simulink model "ATTITUDE_DETERMINATION"  (R2024b)
settings: Solver=VariableStepAuto  StartTime=0.0  StopTime=10.0  RelTol=1e-3
libraries: matrix_library x7
settings Model: Creator=esteb  LastModifiedBy=esteb

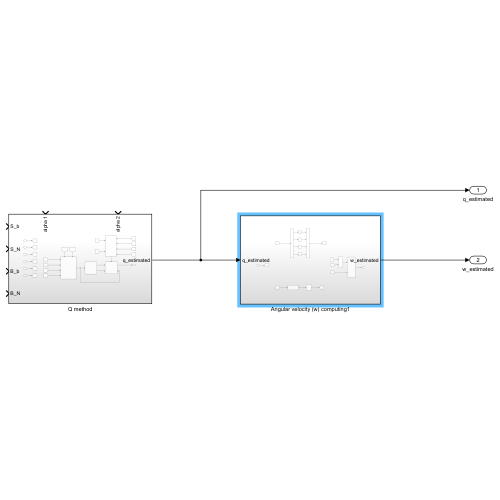
[thumbnail: Simulink's stored preview of the top-level diagram]
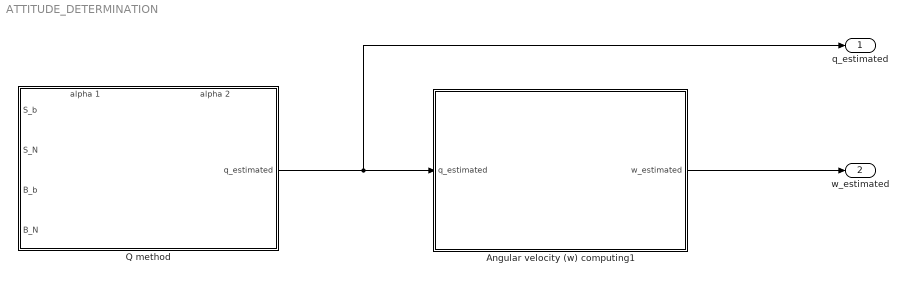
== system ATTITUDE_DETERMINATION ==
  Angular velocity (w) computing1 : Subsystem
  Q method : Subsystem
      settings: PortSchema="{\"entries\":[{\"content\":{\"sides\":[{\"content\":{\"connectorIds\":[\"In1\",\"In2\",\"In3\",\"In4\"]},\"type\":\"ConnectorPlacement.EquallySpacedRectSide\",\"uuid\":\"15956c10-3c30-4cb4-a63c-f434daa5cd48\"},{\"content\":{\"connectorIds\":[\"Out1\"],\"side\":\"RIGHT\"},\"type\":\"ConnectorPlacement.EquallySpacedRectSide\",\"uuid\":\"3f26d307-35c8-43a0-9998-86e1286678fb\"},{\"content\":{\"connectorIds\":[\"In5\",\"In6\"],\"side\":\"TOP\"},\"type\":\"ConnectorPlacement.EquallySpacedRectSide\",\"uuid\":\"55f51305-766e-4e3f-8617-95c7676083b2\"}]},\"type\":\"ConnectorPlacement.EquallySpacedConnector\",\"uuid\":\"09b6cbb7-0430-4316-92af-7ec4423129aa\"}],\"packageUris\":[\"http://schema.mathworks.com/mf0/Connector/R2020b\"],\"version\":\"1.0\"}"
  q_estimated : Outport
  w_estimated : Outport  Port=2
  wires:
  Q method/1(q_estimated) -> Angular velocity (w) computing1/1(q_estimated), q_estimated/1
  Angular velocity (w) computing1/1(w_estimated) -> w_estimated/1

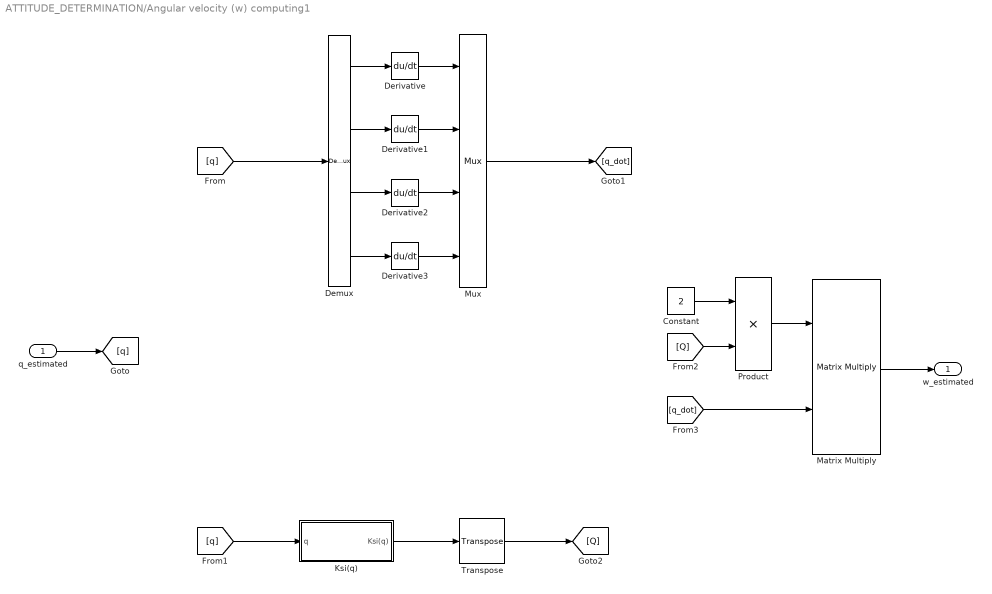
== system ATTITUDE_DETERMINATION/Angular velocity (w) computing1 ==
  q_estimated : Inport
  Constant : Constant  Value=2
  Demux : Demux
  Derivative{,1..3} (4 alike) : Derivative
  Ksi(q) : Subsystem
  Matrix Multiply : Product  Multiplication=Matrix(*)
  Mux : Mux
  Product : Product
  Transpose : matrix_library/Transpose
  w_estimated : Outport
  wires:
  q_estimated/1 -> [q]
  [q] -> Demux/1
  Demux/1 -> Derivative/1
  Demux/2 -> Derivative1/1
  Demux/3 -> Derivative2/1
  Demux/4 -> Derivative3/1
  [q] -> Ksi(q)/1(q)
  Mux/1 -> [q_dot]
  [Q] -> Product/2
  Constant/1 -> Product/1
  [q_dot] -> Matrix Multiply/2
  Matrix Multiply/1 -> w_estimated/1
  Derivative/1 -> Mux/1
  Derivative1/1 -> Mux/2
  Derivative2/1 -> Mux/3
  Derivative3/1 -> Mux/4
  Product/1 -> Matrix Multiply/1
  Ksi(q)/1(Ksi(q)) -> Transpose/1
  Transpose/1 -> [Q]

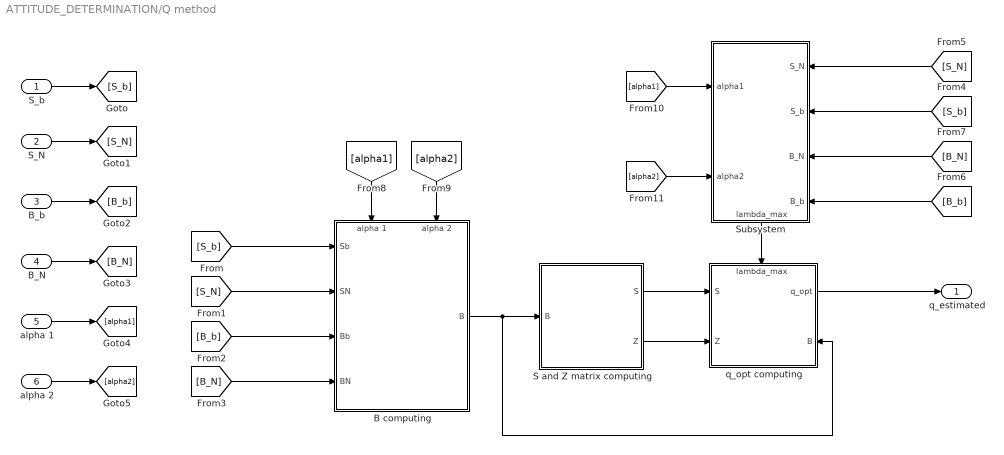
== system ATTITUDE_DETERMINATION/Q method ==
  S_b : Inport
  S_N : Inport  Port=2
  B_b : Inport  Port=3
  B_N : Inport  Port=4
  alpha 1 : Inport  Port=5
  alpha 2 : Inport  Port=6
  B computing : Subsystem
      settings: PortSchema="{\"entries\":[{\"content\":{\"sides\":[{\"content\":{\"connectorIds\":[\"In1\",\"In2\",\"In3\",\"In4\"]},\"type\":\"ConnectorPlacement.EquallySpacedRectSide\",\"uuid\":\"50fc9399-82b5-4b10-921b-f93011029ce3\"},{\"content\":{\"connectorIds\":[\"Out1\"],\"side\":\"RIGHT\"},\"type\":\"ConnectorPlacement.EquallySpacedRectSide\",\"uuid\":\"3981c554-ab38-4f62-9b84-94877d1cd2ff\"},{\"content\":{\"connectorIds\":[\"In5\",\"In6\"],\"side\":\"TOP\"},\"type\":\"ConnectorPlacement.EquallySpacedRectSide\",\"uuid\":\"ba062d99-6f44-4068-8114-c0cfa81f1ff2\"},{\"content\":{\"side\":\"BOTTOM\"},\"type\":\"ConnectorPlacement.EquallySpacedRectSide\",\"uuid\":\"0ce0d8e8-da8b-4b2d-90df-7b0bc851bc5b\"}]},\"type\":\"ConnectorPlacement.EquallySpacedConnector\",\"uuid\":\"bcda7430-c6c8-4f59-a99a-b367d20ffcb5\"}],\"packageUris\":[\"http://schema.mathworks.com/mf0/Connector/R2020b\"],\"version\":\"1.0\"}"
  S and Z matrix computing : Subsystem
  Subsystem : Subsystem
      settings: PortSchema="{\"entries\":[{\"content\":{\"sides\":[{\"content\":{\"connectorIds\":[\"Out1\"]},\"type\":\"ConnectorPlacement.EquallySpacedRectSide\",\"uuid\":\"5768cb62-7f28-4cce-8da1-dcdd14add895\"},{\"content\":{\"side\":\"RIGHT\"},\"type\":\"ConnectorPlacement.EquallySpacedRectSide\",\"uuid\":\"8778aa17-5802-4f6c-9df9-b85455c7c074\"},{\"content\":{\"connectorIds\":[\"In1\",\"In2\"],\"side\":\"TOP\"},\"type\":\"ConnectorPlacement.EquallySpacedRectSide\",\"uuid\":\"8a3cb844-269f-4d3f-b8ee-2af4584390c1\"},{\"content\":{\"connectorIds\":[\"In3\",\"In4\",\"In5\",\"In6\"],\"side\":\"BOTTOM\"},\"type\":\"ConnectorPlacement.EquallySpacedRectSide\",\"uuid\":\"ccc3bad4-265e-44f4-a8b0-aae769a28e60\"}]},\"type\":\"ConnectorPlacement.EquallySpacedConnector\",\"uuid\":\"9389ccda-4d08-49a8-9951-bd9019203c57\"}],\"packageUris\":[\"http://schema.mathworks.com/mf0/Connector/R2020b\"],\"version\":\"1.0\"}"
  q_opt computing : Subsystem
      settings: PortSchema="{\"entries\":[{\"content\":{\"sides\":[{\"content\":{\"connectorIds\":[\"In1\",\"In2\"]},\"type\":\"ConnectorPlacement.EquallySpacedRectSide\",\"uuid\":\"077e0174-8a2c-4f76-bac9-e91df836f5e1\"},{\"content\":{\"connectorIds\":[\"Out1\",\"In4\"],\"side\":\"RIGHT\"},\"type\":\"ConnectorPlacement.EquallySpacedRectSide\",\"uuid\":\"0e923535-8f32-4607-bd4a-42896d211835\"},{\"content\":{\"connectorIds\":[\"In3\"],\"side\":\"TOP\"},\"type\":\"ConnectorPlacement.EquallySpacedRectSide\",\"uuid\":\"91682e2a-1ae8-44b6-9458-d5d75f2c9b10\"},{\"content\":{\"side\":\"BOTTOM\"},\"type\":\"ConnectorPlacement.EquallySpacedRectSide\",\"uuid\":\"ebee2d10-c6a3-420b-a3da-5d4d259a0e4d\"}]},\"type\":\"ConnectorPlacement.EquallySpacedConnector\",\"uuid\":\"6651e596-192f-4f32-9855-13a8c081df01\"}],\"packageUris\":[\"http://schema.mathworks.com/mf0/Connector/R2020b\"],\"version\":\"1.0\"}"
  q_estimated : Outport
  wires:
  [alpha2] -> Subsystem/1(alpha2)
  alpha 1/1 -> [alpha1]
  [B_b] -> B computing/3(Bb)
  S_b/1 -> [S_b]
  [B_N] -> B computing/4(BN)
  [S_N] -> B computing/2(SN)
  B computing/1(B) -> q_opt computing/4(B), S and Z matrix computing/1(B)
  [S_N] -> Subsystem/6(S_N)
  [B_b] -> Subsystem/3(B_b)
  [S_b] -> Subsystem/5(S_b)
  B_N/1 -> [B_N]
  S_N/1 -> [S_N]
  [B_N] -> Subsystem/4(B_N)
  B_b/1 -> [B_b]
  [alpha1] -> Subsystem/2(alpha1)
  [alpha1] -> B computing/5(alpha 1)
  [S_b] -> B computing/1(Sb)
  S and Z matrix computing/1(S) -> q_opt computing/1(S)
  [alpha2] -> B computing/6(alpha 2)
  alpha 2/1 -> [alpha2]
  S and Z matrix computing/2(Z) -> q_opt computing/2(Z)
  Subsystem/1(lambda_max) -> q_opt computing/3(lambda_max)
  q_opt computing/1(q_opt) -> q_estimated/1

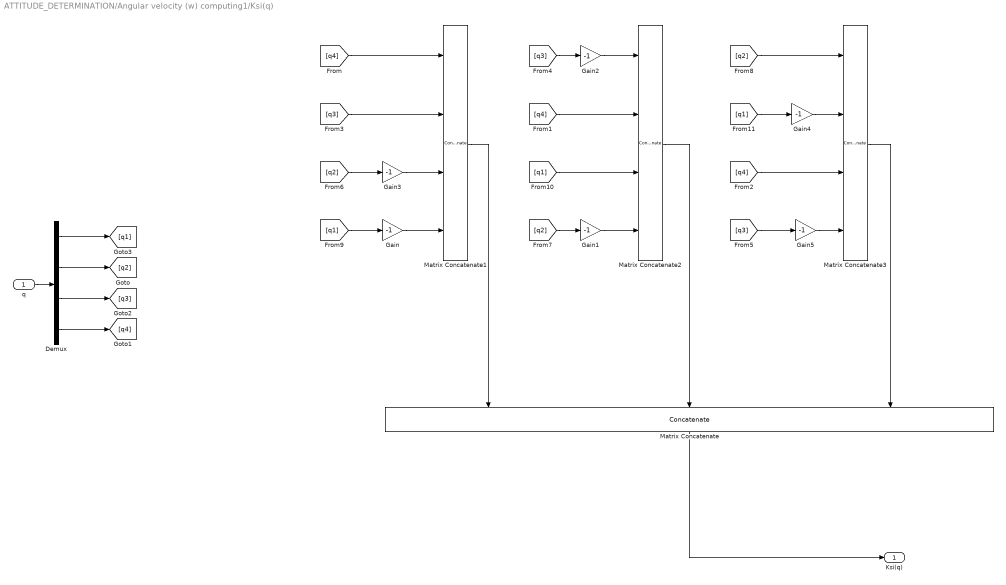
== system ATTITUDE_DETERMINATION/Angular velocity (w) computing1/Ksi(q) ==
  q : Inport
  Demux : Demux
  Gain{,1..5} (6 alike) : Gain  Gain=-1
  Matrix Concatenate : Concatenate  NumInputs=3  Mode=Multidimensional array
  Matrix Concatenate1 : Concatenate  NumInputs=4  Mode=Multidimensional array  ConcatenateDimension=2
  Matrix Concatenate2 : Concatenate  NumInputs=4  Mode=Multidimensional array  ConcatenateDimension=2
  Matrix Concatenate3 : Concatenate  NumInputs=4  Mode=Multidimensional array  ConcatenateDimension=2
  Ksi(q) : Outport
  wires:
  q/1 -> Demux/1
  Demux/2 -> [q2]
  Demux/3 -> [q3]
  Demux/4 -> [q4]
  Demux/1 -> [q1]
  Matrix Concatenate/1 -> Ksi(q)/1
  Matrix Concatenate1/1 -> Matrix Concatenate/1
  Gain1/1 -> Matrix Concatenate2/4
  [q1] -> Matrix Concatenate2/3
  Gain/1 -> Matrix Concatenate1/4
  [q3] -> Matrix Concatenate1/2
  [q2] -> Matrix Concatenate3/1
  Gain5/1 -> Matrix Concatenate3/4
  [q4] -> Matrix Concatenate1/1
  [q4] -> Matrix Concatenate2/2
  [q4] -> Matrix Concatenate3/3
  [q3] -> Gain2/1
  [q3] -> Gain5/1
  [q2] -> Gain3/1
  [q2] -> Gain1/1
  [q1] -> Gain/1
  [q1] -> Gain4/1
  Gain3/1 -> Matrix Concatenate1/3
  Gain2/1 -> Matrix Concatenate2/1
  Gain4/1 -> Matrix Concatenate3/2
  Matrix Concatenate3/1 -> Matrix Concatenate/3
  Matrix Concatenate2/1 -> Matrix Concatenate/2

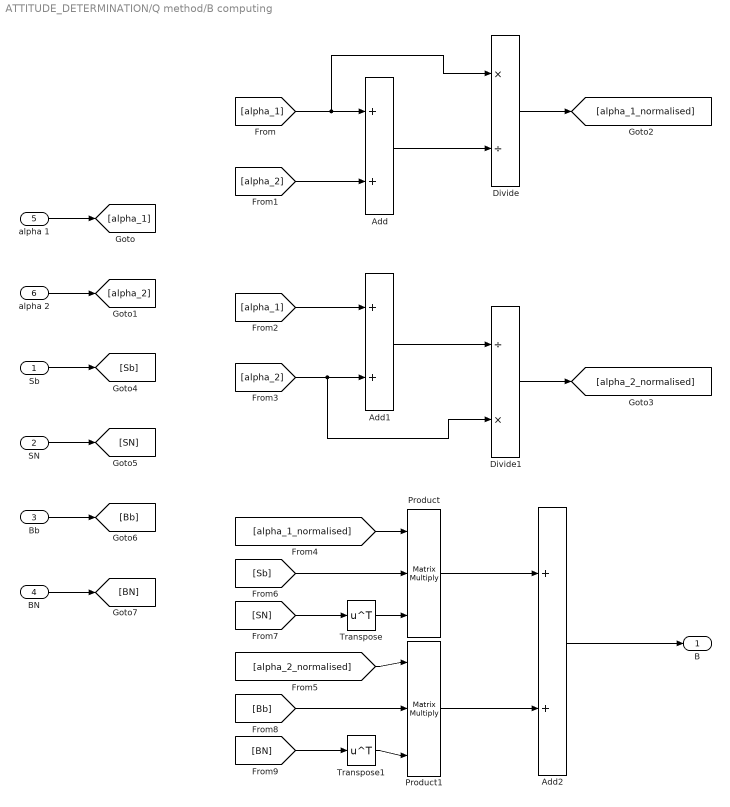
== system ATTITUDE_DETERMINATION/Q method/B computing ==
  Sb : Inport
  SN : Inport  Port=2
  Bb : Inport  Port=3
  BN : Inport  Port=4
  alpha 1 : Inport  Port=5
  alpha 2 : Inport  Port=6
  Add : Sum
  Add1 : Sum
  Add2 : Sum
  Divide : Product  Inputs=*/
  Divide1 : Product  Inputs=/*
  Product : Product  Inputs=3  Multiplication=Matrix(*)
  Product1 : Product  Inputs=3  Multiplication=Matrix(*)
  Transpose : Math  Operator=transpose
  Transpose1 : Math  Operator=transpose
  B : Outport
  wires:
  alpha 1/1 -> [alpha_1]
  alpha 2/1 -> [alpha_2]
  [alpha_1] -> Divide/1, Add/1
  [alpha_2] -> Add/2
  Add/1 -> Divide/2
  Divide/1 -> [alpha_1_normalised]
  [alpha_2] -> Divide1/2, Add1/2
  Divide1/1 -> [alpha_2_normalised]
  [alpha_1] -> Add1/1
  Add1/1 -> Divide1/1
  SN/1 -> [SN]
  Sb/1 -> [Sb]
  Bb/1 -> [Bb]
  BN/1 -> [BN]
  Product/1 -> Add2/1
  Product1/1 -> Add2/2
  [alpha_1_normalised] -> Product/1
  [alpha_2_normalised] -> Product1/1
  [Sb] -> Product/2
  Transpose/1 -> Product/3
  Transpose1/1 -> Product1/3
  [SN] -> Transpose/1
  [Bb] -> Product1/2
  [BN] -> Transpose1/1
  Add2/1 -> B/1

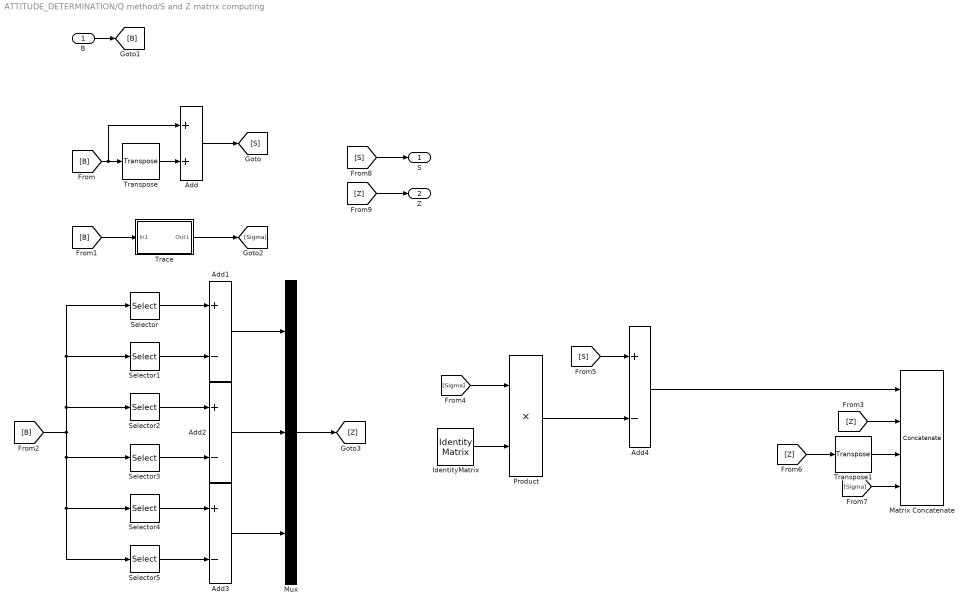
== system ATTITUDE_DETERMINATION/Q method/S and Z matrix computing ==
  B : Inport
  Add : Sum
  Add{1..4} (4 alike) : Sum  Inputs=+-
  IdentityMatrix : IdentityMatrix
  Matrix Concatenate : Concatenate  NumInputs=4  Mode=Multidimensional array  ConcatenateDimension=2
  Mux : Mux  Inputs=3
  Product : Product
  Selector : Selector  NumberOfDimensions=2  InputPortWidth=3  IndexOptions=Index vector (dialog),Index vector (dialog)  Indices=2,3  OutputSizes=1,1
  Selector1 : Selector  NumberOfDimensions=2  InputPortWidth=3  IndexOptions=Index vector (dialog),Index vector (dialog)  Indices=3,2  OutputSizes=1,1
  Selector2 : Selector  NumberOfDimensions=2  InputPortWidth=3  IndexOptions=Index vector (dialog),Index vector (dialog)  Indices=3,1  OutputSizes=1,1
  Selector3 : Selector  NumberOfDimensions=2  InputPortWidth=3  IndexOptions=Index vector (dialog),Index vector (dialog)  Indices=1,3  OutputSizes=1,1
  Selector4 : Selector  NumberOfDimensions=2  InputPortWidth=3  IndexOptions=Index vector (dialog),Index vector (dialog)  Indices=1,2  OutputSizes=1,1
  Selector5 : Selector  NumberOfDimensions=2  InputPortWidth=3  IndexOptions=Index vector (dialog),Index vector (dialog)  Indices=2,1  OutputSizes=1,1
  Trace : Subsystem
  Transpose : matrix_library/Transpose
  Transpose1 : matrix_library/Transpose
  S : Outport
  Z : Outport  Port=2
  wires:
  [B] -> Add/1, Transpose/1
  Transpose/1 -> Add/2
  Add/1 -> [S]
  B/1 -> [B]
  [B] -> Trace/1(In1)
  Trace/1(Out1) -> [Sigma]
  [B] -> Selector/1, Selector1/1, Selector2/1, Selector5/1, Selector4/1, Selector3/1
  Selector/1 -> Add1/1
  Selector1/1 -> Add1/2
  Selector4/1 -> Add3/1
  Selector5/1 -> Add3/2
  Selector3/1 -> Add2/2
  Selector2/1 -> Add2/1
  Add1/1 -> Mux/1
  Add2/1 -> Mux/2
  Add3/1 -> Mux/3
  Mux/1 -> [Z]
  [Z] -> Matrix Concatenate/2
  [Sigma] -> Product/1
  IdentityMatrix/1 -> Product/2
  Product/1 -> Add4/2
  [S] -> Add4/1
  Add4/1 -> Matrix Concatenate/1
  Transpose1/1 -> Matrix Concatenate/3
  [Z] -> Transpose1/1
  [Sigma] -> Matrix Concatenate/4
  [S] -> S/1
  [Z] -> Z/1

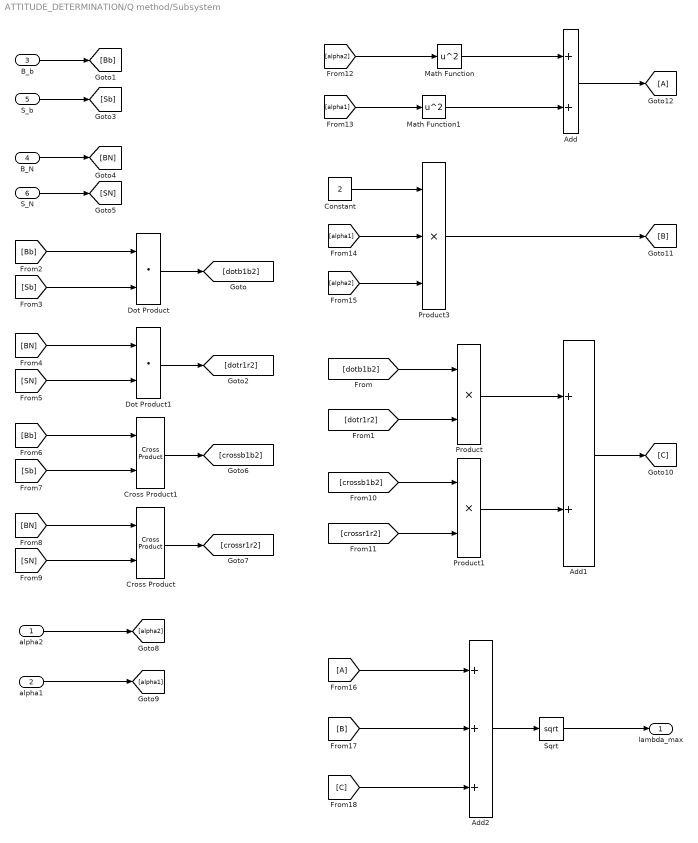
== system ATTITUDE_DETERMINATION/Q method/Subsystem ==
  alpha2 : Inport
  alpha1 : Inport  Port=2
  B_b : Inport  Port=3
  B_N : Inport  Port=4
  S_b : Inport  Port=5
  S_N : Inport  Port=6
  Add : Sum
  Add1 : Sum
  Add2 : Sum  Inputs=+++
  Constant : Constant  Value=2
  Cross Product : matrix_library/Cross Product
  Cross Product1 : matrix_library/Cross Product
  Dot Product : DotProduct  OutDataTypeStr=Inherit: Inherit via internal rule
  Dot Product1 : DotProduct  OutDataTypeStr=Inherit: Inherit via internal rule
  From16 : From
  Goto12 : Goto
  Math Function : Math  Operator=square
  Math Function1 : Math  Operator=square
  Product : Product
  Product1 : Product
  Product3 : Product  Inputs=3
  Sqrt : Sqrt
  lambda_max : Outport
  wires:
  Math Function/1 -> Add/1
  Math Function1/1 -> Add/2
  Dot Product/1 -> [dotb1b2]
  Dot Product1/1 -> [dotr1r2]
  [dotr1r2] -> Product/2
  [dotb1b2] -> Product/1
  B_b/1 -> [Bb]
  S_b/1 -> [Sb]
  B_N/1 -> [BN]
  S_N/1 -> [SN]
  [Sb] -> Dot Product/2
  [Bb] -> Dot Product/1
  [SN] -> Dot Product1/2
  [BN] -> Dot Product1/1
  [Bb] -> Cross Product1/1
  [Sb] -> Cross Product1/2
  [BN] -> Cross Product/1
  [SN] -> Cross Product/2
  Cross Product1/1 -> [crossb1b2]
  Cross Product/1 -> [crossr1r2]
  [crossb1b2] -> Product1/1
  [crossr1r2] -> Product1/2
  Product1/1 -> Add1/2
  Product/1 -> Add1/1
  alpha2/1 -> [alpha2]
  alpha1/1 -> [alpha1]
  [alpha2] -> Math Function/1
  [alpha1] -> Math Function1/1
  [alpha2] -> Product3/3
  [alpha1] -> Product3/2
  Constant/1 -> Product3/1
  Add1/1 -> [C]
  Product3/1 -> [B]
  Add/1 -> Goto12/1
  [C] -> Add2/3
  [B] -> Add2/2
  From16/1 -> Add2/1
  Add2/1 -> Sqrt/1
  Sqrt/1 -> lambda_max/1

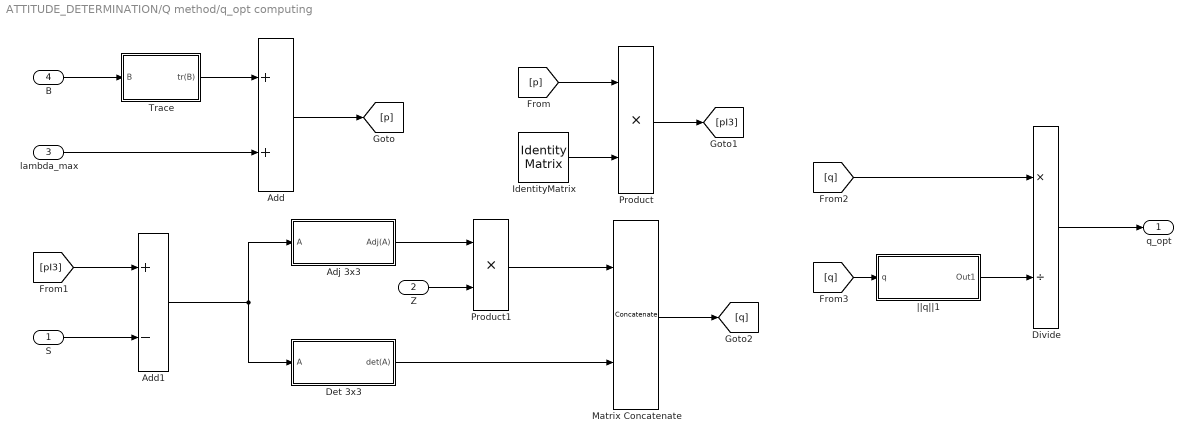
== system ATTITUDE_DETERMINATION/Q method/q_opt computing ==
  S : Inport
  Z : Inport  Port=2
  lambda_max : Inport  Port=3
  B : Inport  Port=4
  Add : Sum
  Add1 : Sum  Inputs=+-
  Adj 3x3 : Subsystem
  Det 3x3 : Subsystem
  Divide : Product  Inputs=*/
  IdentityMatrix : IdentityMatrix
  Matrix Concatenate : Concatenate  Mode=Multidimensional array
  Product : Product
  Product1 : Product
  Trace : Subsystem
  ||q||1 : Subsystem
  q_opt : Outport
  wires:
  B/1 -> Trace/1(B)
  lambda_max/1 -> Add/2
  Trace/1(tr(B)) -> Add/1
  Add/1 -> [p]
  IdentityMatrix/1 -> Product/2
  [p] -> Product/1
  Product/1 -> [pI3]
  S/1 -> Add1/2
  [pI3] -> Add1/1
  Add1/1 -> Det 3x3/1(A), Adj 3x3/1(A)
  Matrix Concatenate/1 -> [q]
  [q] -> Divide/1
  [q] -> ||q||1/1(q)
  Divide/1 -> q_opt/1
  Z/1 -> Product1/2
  Adj 3x3/1(Adj(A)) -> Product1/1
  Product1/1 -> Matrix Concatenate/1
  Det 3x3/1(det(A)) -> Matrix Concatenate/2
  ||q||1/1(Out1) -> Divide/2

== system ATTITUDE_DETERMINATION/Q method/S and Z matrix computing/Trace ==
  In1 : Inport
  Extract Diagonal : matrix_library/Extract Diagonal
  Sum of Elements : Sum  Inputs=+
  Out1 : Outport
  wires:
  In1/1 -> Extract Diagonal/1
  Extract Diagonal/1 -> Sum of Elements/1
  Sum of Elements/1 -> Out1/1

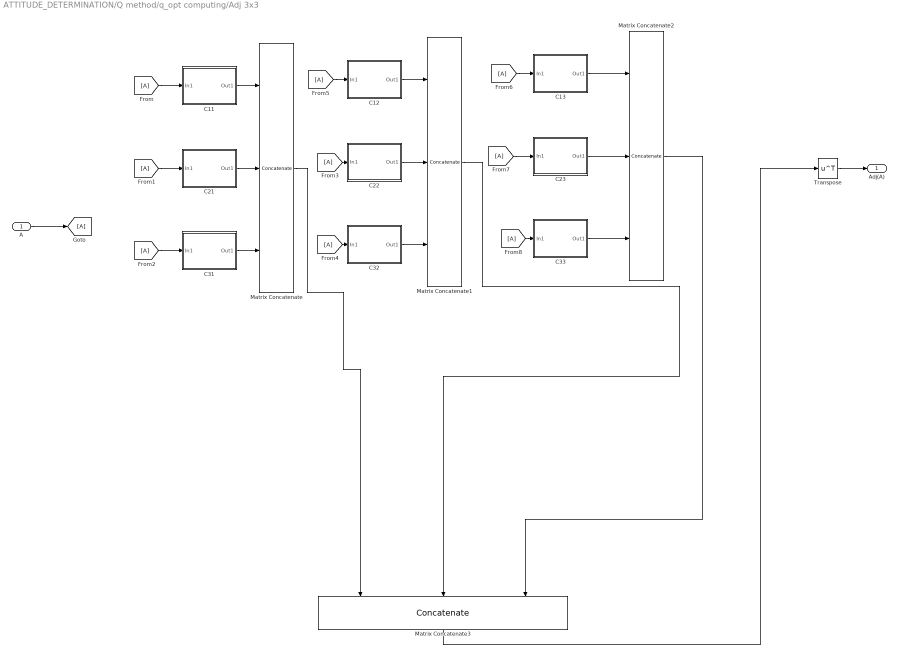
== system ATTITUDE_DETERMINATION/Q method/q_opt computing/Adj 3x3 ==
  A : Inport
  C11 : Subsystem
  C12 : Subsystem
  C13 : Subsystem
  C21 : Subsystem
  C22 : Subsystem
  C23 : Subsystem
  C31 : Subsystem
  C32 : Subsystem
  C33 : Subsystem
  From{,1..8} (9 alike) : From
  Goto : Goto
  Matrix Concatenate : Concatenate  NumInputs=3  Mode=Multidimensional array
  Matrix Concatenate1 : Concatenate  NumInputs=3  Mode=Multidimensional array
  Matrix Concatenate2 : Concatenate  NumInputs=3  Mode=Multidimensional array
  Matrix Concatenate3 : Concatenate  NumInputs=3  Mode=Multidimensional array  ConcatenateDimension=2
  Transpose : Math  Operator=transpose
  Adj(A) : Outport
  wires:
  Transpose/1 -> Adj(A)/1
  A/1 -> Goto/1
  C11/1(Out1) -> Matrix Concatenate/1
  C21/1(Out1) -> Matrix Concatenate/2
  C31/1(Out1) -> Matrix Concatenate/3
  C22/1(Out1) -> Matrix Concatenate1/2
  C12/1(Out1) -> Matrix Concatenate1/1
  C32/1(Out1) -> Matrix Concatenate1/3
  C23/1(Out1) -> Matrix Concatenate2/2
  C13/1(Out1) -> Matrix Concatenate2/1
  C33/1(Out1) -> Matrix Concatenate2/3
  Matrix Concatenate3/1 -> Transpose/1
  Matrix Concatenate2/1 -> Matrix Concatenate3/3
  Matrix Concatenate1/1 -> Matrix Concatenate3/2
  Matrix Concatenate/1 -> Matrix Concatenate3/1
  From/1 -> C11/1(In1)
  From1/1 -> C21/1(In1)
  From2/1 -> C31/1(In1)
  From3/1 -> C22/1(In1)
  From4/1 -> C32/1(In1)
  From5/1 -> C12/1(In1)
  From6/1 -> C13/1(In1)
  From7/1 -> C23/1(In1)
  From8/1 -> C33/1(In1)

== system ATTITUDE_DETERMINATION/Q method/q_opt computing/Det 3x3 ==
  A : Inport
  Adj 3x3 : Subsystem
  Matrix Multiply : Product  Multiplication=Matrix(*)
  Selector : Selector  NumberOfDimensions=2  InputPortWidth=3  IndexOptions=Index vector (dialog),Index vector (dialog)  Indices=1,1  OutputSizes=1,1
  det(A) : Outport
  wires:
  A/1 -> Adj 3x3/1(In1), Matrix Multiply/1
  Adj 3x3/1(Out1) -> Matrix Multiply/2
  Matrix Multiply/1 -> Selector/1
  Selector/1 -> det(A)/1

== system ATTITUDE_DETERMINATION/Q method/q_opt computing/Trace ==
  B : Inport
  Extract Diagonal : matrix_library/Extract Diagonal
  Sum of Elements : Sum  Inputs=+
  tr(B) : Outport
  wires:
  B/1 -> Extract Diagonal/1
  Extract Diagonal/1 -> Sum of Elements/1
  Sum of Elements/1 -> tr(B)/1

== system ATTITUDE_DETERMINATION/Q method/q_opt computing/||q||1 ==
  q : Inport
  MatrixMultiply : Product  Multiplication=Matrix(*)
  Selector : Selector  NumberOfDimensions=2  InputPortWidth=3  IndexOptions=Index vector (dialog),Index vector (dialog)  Indices=1,1  OutputSizes=1,1
  Sqrt : Sqrt
  "[q (x)]" : Subsystem
  q* : Subsystem
  Out1 : Outport
  wires:
  q/1 -> "[q (x)]"/1(In1), q*/1(q)
  q*/1(q*) -> MatrixMultiply/2
  "[q (x)]"/1(Out1) -> MatrixMultiply/1
  MatrixMultiply/1 -> Selector/1
  Selector/1 -> Sqrt/1
  Sqrt/1 -> Out1/1

== system ATTITUDE_DETERMINATION/Q method/q_opt computing/Adj 3x3/C11 ==
  In1 : Inport
  22 : Selector  NumberOfDimensions=2  InputPortWidth=3  IndexOptions=Index vector (dialog),Index vector (dialog)  Indices=2,2  OutputSizes=1,1
  23 : Selector  NumberOfDimensions=2  InputPortWidth=3  IndexOptions=Index vector (dialog),Index vector (dialog)  Indices=2,3  OutputSizes=1,1
  32 : Selector  NumberOfDimensions=2  InputPortWidth=3  IndexOptions=Index vector (dialog),Index vector (dialog)  Indices=3,2  OutputSizes=1,1
  33 : Selector  NumberOfDimensions=2  InputPortWidth=3  IndexOptions=Index vector (dialog),Index vector (dialog)  Indices=3,3  OutputSizes=1,1
  Product : Product
  Product1 : Product
  Subtract : Sum  Inputs=+-
  Out1 : Outport
  wires:
  In1/1 -> 32/1, 23/1, 33/1, 22/1
  22/1 -> Product/1
  33/1 -> Product/2
  23/1 -> Product1/1
  32/1 -> Product1/2
  Subtract/1 -> Out1/1
  Product/1 -> Subtract/1
  Product1/1 -> Subtract/2

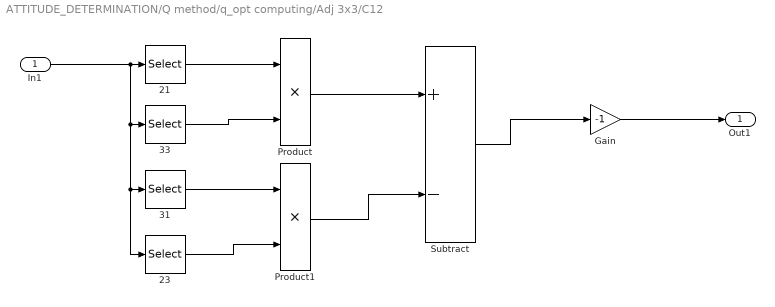
== system ATTITUDE_DETERMINATION/Q method/q_opt computing/Adj 3x3/C12 ==
  In1 : Inport
  21 : Selector  NumberOfDimensions=2  InputPortWidth=3  IndexOptions=Index vector (dialog),Index vector (dialog)  Indices=2,1  OutputSizes=1,1
  23 : Selector  NumberOfDimensions=2  InputPortWidth=3  IndexOptions=Index vector (dialog),Index vector (dialog)  Indices=2,3  OutputSizes=1,1
  31 : Selector  NumberOfDimensions=2  InputPortWidth=3  IndexOptions=Index vector (dialog),Index vector (dialog)  Indices=3,1  OutputSizes=1,1
  33 : Selector  NumberOfDimensions=2  InputPortWidth=3  IndexOptions=Index vector (dialog),Index vector (dialog)  Indices=3,3  OutputSizes=1,1
  Gain : Gain  Gain=-1
  Product : Product
  Product1 : Product
  Subtract : Sum  Inputs=+-
  Out1 : Outport
  wires:
  In1/1 -> 23/1, 31/1, 33/1, 21/1
  21/1 -> Product/1
  33/1 -> Product/2
  31/1 -> Product1/1
  23/1 -> Product1/2
  Subtract/1 -> Gain/1
  Product/1 -> Subtract/1
  Product1/1 -> Subtract/2
  Gain/1 -> Out1/1

== system ATTITUDE_DETERMINATION/Q method/q_opt computing/Adj 3x3/C13 ==
  In1 : Inport
  21 : Selector  NumberOfDimensions=2  InputPortWidth=3  IndexOptions=Index vector (dialog),Index vector (dialog)  Indices=2,1  OutputSizes=1,1
  22 : Selector  NumberOfDimensions=2  InputPortWidth=3  IndexOptions=Index vector (dialog),Index vector (dialog)  Indices=2,2  OutputSizes=1,1
  31 : Selector  NumberOfDimensions=2  InputPortWidth=3  IndexOptions=Index vector (dialog),Index vector (dialog)  Indices=3,1  OutputSizes=1,1
  32 : Selector  NumberOfDimensions=2  InputPortWidth=3  IndexOptions=Index vector (dialog),Index vector (dialog)  Indices=3,2  OutputSizes=1,1
  Product : Product
  Product1 : Product
  Subtract : Sum  Inputs=+-
  Out1 : Outport
  wires:
  In1/1 -> 31/1, 22/1, 32/1, 21/1
  21/1 -> Product/1
  32/1 -> Product/2
  22/1 -> Product1/1
  31/1 -> Product1/2
  Subtract/1 -> Out1/1
  Product/1 -> Subtract/1
  Product1/1 -> Subtract/2

== system ATTITUDE_DETERMINATION/Q method/q_opt computing/Adj 3x3/C21 ==
  In1 : Inport
  12 : Selector  NumberOfDimensions=2  InputPortWidth=3  IndexOptions=Index vector (dialog),Index vector (dialog)  Indices=1,2  OutputSizes=1,1
  13 : Selector  NumberOfDimensions=2  InputPortWidth=3  IndexOptions=Index vector (dialog),Index vector (dialog)  Indices=1,3  OutputSizes=1,1
  32 : Selector  NumberOfDimensions=2  InputPortWidth=3  IndexOptions=Index vector (dialog),Index vector (dialog)  Indices=3,2  OutputSizes=1,1
  33 : Selector  NumberOfDimensions=2  InputPortWidth=3  IndexOptions=Index vector (dialog),Index vector (dialog)  Indices=3,3  OutputSizes=1,1
  Gain : Gain  Gain=-1
  Product : Product
  Product1 : Product
  Subtract : Sum  Inputs=+-
  Out1 : Outport
  wires:
  In1/1 -> 32/1, 13/1, 33/1, 12/1
  12/1 -> Product/1
  33/1 -> Product/2
  13/1 -> Product1/1
  32/1 -> Product1/2
  Subtract/1 -> Gain/1
  Product/1 -> Subtract/1
  Product1/1 -> Subtract/2
  Gain/1 -> Out1/1

== system ATTITUDE_DETERMINATION/Q method/q_opt computing/Adj 3x3/C22 ==
  In1 : Inport
  11 : Selector  NumberOfDimensions=2  InputPortWidth=3  IndexOptions=Index vector (dialog),Index vector (dialog)  Indices=1,1  OutputSizes=1,1
  13 : Selector  NumberOfDimensions=2  InputPortWidth=3  IndexOptions=Index vector (dialog),Index vector (dialog)  Indices=1,3  OutputSizes=1,1
  31 : Selector  NumberOfDimensions=2  InputPortWidth=3  IndexOptions=Index vector (dialog),Index vector (dialog)  Indices=3,1  OutputSizes=1,1
  33 : Selector  NumberOfDimensions=2  InputPortWidth=3  IndexOptions=Index vector (dialog),Index vector (dialog)  Indices=3,3  OutputSizes=1,1
  Product : Product
  Product1 : Product
  Subtract : Sum  Inputs=+-
  Out1 : Outport
  wires:
  In1/1 -> 31/1, 13/1, 33/1, 11/1
  11/1 -> Product/1
  33/1 -> Product/2
  13/1 -> Product1/1
  31/1 -> Product1/2
  Subtract/1 -> Out1/1
  Product/1 -> Subtract/1
  Product1/1 -> Subtract/2

== system ATTITUDE_DETERMINATION/Q method/q_opt computing/Adj 3x3/C23 ==
  In1 : Inport
  11 : Selector  NumberOfDimensions=2  InputPortWidth=3  IndexOptions=Index vector (dialog),Index vector (dialog)  Indices=1,1  OutputSizes=1,1
  12 : Selector  NumberOfDimensions=2  InputPortWidth=3  IndexOptions=Index vector (dialog),Index vector (dialog)  Indices=1,2  OutputSizes=1,1
  31 : Selector  NumberOfDimensions=2  InputPortWidth=3  IndexOptions=Index vector (dialog),Index vector (dialog)  Indices=3,1  OutputSizes=1,1
  32 : Selector  NumberOfDimensions=2  InputPortWidth=3  IndexOptions=Index vector (dialog),Index vector (dialog)  Indices=3,2  OutputSizes=1,1
  Gain : Gain  Gain=-1
  Product : Product
  Product1 : Product
  Subtract : Sum  Inputs=+-
  Out1 : Outport
  wires:
  In1/1 -> 12/1, 31/1, 32/1, 11/1
  11/1 -> Product/1
  32/1 -> Product/2
  31/1 -> Product1/1
  12/1 -> Product1/2
  Subtract/1 -> Gain/1
  Product/1 -> Subtract/1
  Product1/1 -> Subtract/2
  Gain/1 -> Out1/1

== system ATTITUDE_DETERMINATION/Q method/q_opt computing/Adj 3x3/C31 ==
  In1 : Inport
  12 : Selector  NumberOfDimensions=2  InputPortWidth=3  IndexOptions=Index vector (dialog),Index vector (dialog)  Indices=1,2  OutputSizes=1,1
  13 : Selector  NumberOfDimensions=2  InputPortWidth=3  IndexOptions=Index vector (dialog),Index vector (dialog)  Indices=1,3  OutputSizes=1,1
  22 : Selector  NumberOfDimensions=2  InputPortWidth=3  IndexOptions=Index vector (dialog),Index vector (dialog)  Indices=2,2  OutputSizes=1,1
  23 : Selector  NumberOfDimensions=2  InputPortWidth=3  IndexOptions=Index vector (dialog),Index vector (dialog)  Indices=2,3  OutputSizes=1,1
  Product : Product
  Product1 : Product
  Subtract : Sum  Inputs=+-
  Out1 : Outport
  wires:
  In1/1 -> 22/1, 13/1, 23/1, 12/1
  12/1 -> Product/1
  23/1 -> Product/2
  13/1 -> Product1/1
  22/1 -> Product1/2
  Subtract/1 -> Out1/1
  Product/1 -> Subtract/1
  Product1/1 -> Subtract/2

== system ATTITUDE_DETERMINATION/Q method/q_opt computing/Adj 3x3/C32 ==
  In1 : Inport
  11 : Selector  NumberOfDimensions=2  InputPortWidth=3  IndexOptions=Index vector (dialog),Index vector (dialog)  Indices=1,1  OutputSizes=1,1
  13 : Selector  NumberOfDimensions=2  InputPortWidth=3  IndexOptions=Index vector (dialog),Index vector (dialog)  Indices=1,3  OutputSizes=1,1
  23 : Selector  NumberOfDimensions=2  InputPortWidth=3  IndexOptions=Index vector (dialog),Index vector (dialog)  Indices=2,3  OutputSizes=1,1
  31 : Selector  NumberOfDimensions=2  InputPortWidth=3  IndexOptions=Index vector (dialog),Index vector (dialog)  Indices=3,1  OutputSizes=1,1
  Gain : Gain  Gain=-1
  Product : Product
  Product1 : Product
  Subtract : Sum  Inputs=+-
  Out1 : Outport
  wires:
  In1/1 -> 31/1, 13/1, 23/1, 11/1
  11/1 -> Product/1
  23/1 -> Product/2
  13/1 -> Product1/1
  31/1 -> Product1/2
  Subtract/1 -> Gain/1
  Product/1 -> Subtract/1
  Product1/1 -> Subtract/2
  Gain/1 -> Out1/1

== system ATTITUDE_DETERMINATION/Q method/q_opt computing/Adj 3x3/C33 ==
  In1 : Inport
  11 : Selector  NumberOfDimensions=2  InputPortWidth=3  IndexOptions=Index vector (dialog),Index vector (dialog)  Indices=1,1  OutputSizes=1,1
  12 : Selector  NumberOfDimensions=2  InputPortWidth=3  IndexOptions=Index vector (dialog),Index vector (dialog)  Indices=1,2  OutputSizes=1,1
  21 : Selector  NumberOfDimensions=2  InputPortWidth=3  IndexOptions=Index vector (dialog),Index vector (dialog)  Indices=2,1  OutputSizes=1,1
  22 : Selector  NumberOfDimensions=2  InputPortWidth=3  IndexOptions=Index vector (dialog),Index vector (dialog)  Indices=2,2  OutputSizes=1,1
  Product : Product
  Product1 : Product
  Subtract : Sum  Inputs=+-
  Out1 : Outport
  wires:
  In1/1 -> 21/1, 12/1, 22/1, 11/1
  11/1 -> Product/1
  22/1 -> Product/2
  12/1 -> Product1/1
  21/1 -> Product1/2
  Subtract/1 -> Out1/1
  Product/1 -> Subtract/1
  Product1/1 -> Subtract/2

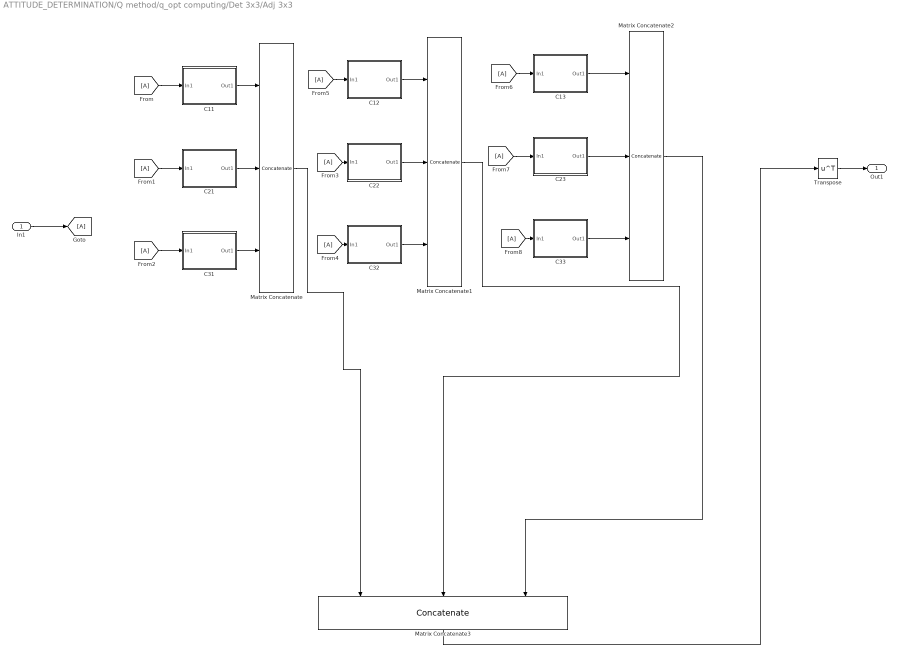
== system ATTITUDE_DETERMINATION/Q method/q_opt computing/Det 3x3/Adj 3x3 ==
  In1 : Inport
  C11 : Subsystem
  C12 : Subsystem
  C13 : Subsystem
  C21 : Subsystem
  C22 : Subsystem
  C23 : Subsystem
  C31 : Subsystem
  C32 : Subsystem
  C33 : Subsystem
  From{,1..8} (9 alike) : From
  Goto : Goto
  Matrix Concatenate : Concatenate  NumInputs=3  Mode=Multidimensional array
  Matrix Concatenate1 : Concatenate  NumInputs=3  Mode=Multidimensional array
  Matrix Concatenate2 : Concatenate  NumInputs=3  Mode=Multidimensional array
  Matrix Concatenate3 : Concatenate  NumInputs=3  Mode=Multidimensional array  ConcatenateDimension=2
  Transpose : Math  Operator=transpose
  Out1 : Outport
  wires:
  Transpose/1 -> Out1/1
  In1/1 -> Goto/1
  C11/1(Out1) -> Matrix Concatenate/1
  C21/1(Out1) -> Matrix Concatenate/2
  C31/1(Out1) -> Matrix Concatenate/3
  C22/1(Out1) -> Matrix Concatenate1/2
  C12/1(Out1) -> Matrix Concatenate1/1
  C32/1(Out1) -> Matrix Concatenate1/3
  C23/1(Out1) -> Matrix Concatenate2/2
  C13/1(Out1) -> Matrix Concatenate2/1
  C33/1(Out1) -> Matrix Concatenate2/3
  Matrix Concatenate3/1 -> Transpose/1
  Matrix Concatenate2/1 -> Matrix Concatenate3/3
  Matrix Concatenate1/1 -> Matrix Concatenate3/2
  Matrix Concatenate/1 -> Matrix Concatenate3/1
  From/1 -> C11/1(In1)
  From1/1 -> C21/1(In1)
  From2/1 -> C31/1(In1)
  From3/1 -> C22/1(In1)
  From4/1 -> C32/1(In1)
  From5/1 -> C12/1(In1)
  From6/1 -> C13/1(In1)
  From7/1 -> C23/1(In1)
  From8/1 -> C33/1(In1)

== system ATTITUDE_DETERMINATION/Q method/q_opt computing/||q||1/[q (x)] ==
  In1 : Inport
  Matrix Concatenate : Concatenate  Mode=Multidimensional array  ConcatenateDimension=2
  Psi(q) : Subsystem
  Out1 : Outport
  wires:
  Psi(q)/1(Out1) -> Matrix Concatenate/1
  In1/1 -> Matrix Concatenate/2, Psi(q)/1(In1)
  Matrix Concatenate/1 -> Out1/1

== system ATTITUDE_DETERMINATION/Q method/q_opt computing/||q||1/q* ==
  note: Evaluate the quaternion coniugate
  q : Inport
  Demux : Demux
  Gain : Gain  Gain=-1
  Gain1 : Gain  Gain=-1
  Gain2 : Gain  Gain=-1
  Mux : Mux
  q* : Outport
  wires:
  Gain2/1 -> Mux/3
  Gain1/1 -> Mux/2
  Gain/1 -> Mux/1
  Demux/3 -> Gain2/1
  Demux/2 -> Gain1/1
  Demux/1 -> Gain/1
  q/1 -> Demux/1
  Demux/4 -> Mux/4
  Mux/1 -> q*/1

== system ATTITUDE_DETERMINATION/Q method/q_opt computing/Det 3x3/Adj 3x3/C11 ==
  In1 : Inport
  22 : Selector  NumberOfDimensions=2  InputPortWidth=3  IndexOptions=Index vector (dialog),Index vector (dialog)  Indices=2,2  OutputSizes=1,1
  23 : Selector  NumberOfDimensions=2  InputPortWidth=3  IndexOptions=Index vector (dialog),Index vector (dialog)  Indices=2,3  OutputSizes=1,1
  32 : Selector  NumberOfDimensions=2  InputPortWidth=3  IndexOptions=Index vector (dialog),Index vector (dialog)  Indices=3,2  OutputSizes=1,1
  33 : Selector  NumberOfDimensions=2  InputPortWidth=3  IndexOptions=Index vector (dialog),Index vector (dialog)  Indices=3,3  OutputSizes=1,1
  Product : Product
  Product1 : Product
  Subtract : Sum  Inputs=+-
  Out1 : Outport
  wires:
  In1/1 -> 32/1, 23/1, 33/1, 22/1
  22/1 -> Product/1
  33/1 -> Product/2
  23/1 -> Product1/1
  32/1 -> Product1/2
  Subtract/1 -> Out1/1
  Product/1 -> Subtract/1
  Product1/1 -> Subtract/2

== system ATTITUDE_DETERMINATION/Q method/q_opt computing/Det 3x3/Adj 3x3/C12 ==
  In1 : Inport
  21 : Selector  NumberOfDimensions=2  InputPortWidth=3  IndexOptions=Index vector (dialog),Index vector (dialog)  Indices=2,1  OutputSizes=1,1
  23 : Selector  NumberOfDimensions=2  InputPortWidth=3  IndexOptions=Index vector (dialog),Index vector (dialog)  Indices=2,3  OutputSizes=1,1
  31 : Selector  NumberOfDimensions=2  InputPortWidth=3  IndexOptions=Index vector (dialog),Index vector (dialog)  Indices=3,1  OutputSizes=1,1
  33 : Selector  NumberOfDimensions=2  InputPortWidth=3  IndexOptions=Index vector (dialog),Index vector (dialog)  Indices=3,3  OutputSizes=1,1
  Gain : Gain  Gain=-1
  Product : Product
  Product1 : Product
  Subtract : Sum  Inputs=+-
  Out1 : Outport
  wires:
  In1/1 -> 23/1, 31/1, 33/1, 21/1
  21/1 -> Product/1
  33/1 -> Product/2
  31/1 -> Product1/1
  23/1 -> Product1/2
  Subtract/1 -> Gain/1
  Product/1 -> Subtract/1
  Product1/1 -> Subtract/2
  Gain/1 -> Out1/1

== system ATTITUDE_DETERMINATION/Q method/q_opt computing/Det 3x3/Adj 3x3/C13 ==
  In1 : Inport
  21 : Selector  NumberOfDimensions=2  InputPortWidth=3  IndexOptions=Index vector (dialog),Index vector (dialog)  Indices=2,1  OutputSizes=1,1
  22 : Selector  NumberOfDimensions=2  InputPortWidth=3  IndexOptions=Index vector (dialog),Index vector (dialog)  Indices=2,2  OutputSizes=1,1
  31 : Selector  NumberOfDimensions=2  InputPortWidth=3  IndexOptions=Index vector (dialog),Index vector (dialog)  Indices=3,1  OutputSizes=1,1
  32 : Selector  NumberOfDimensions=2  InputPortWidth=3  IndexOptions=Index vector (dialog),Index vector (dialog)  Indices=3,2  OutputSizes=1,1
  Product : Product
  Product1 : Product
  Subtract : Sum  Inputs=+-
  Out1 : Outport
  wires:
  In1/1 -> 31/1, 22/1, 32/1, 21/1
  21/1 -> Product/1
  32/1 -> Product/2
  22/1 -> Product1/1
  31/1 -> Product1/2
  Subtract/1 -> Out1/1
  Product/1 -> Subtract/1
  Product1/1 -> Subtract/2

== system ATTITUDE_DETERMINATION/Q method/q_opt computing/Det 3x3/Adj 3x3/C21 ==
  In1 : Inport
  12 : Selector  NumberOfDimensions=2  InputPortWidth=3  IndexOptions=Index vector (dialog),Index vector (dialog)  Indices=1,2  OutputSizes=1,1
  13 : Selector  NumberOfDimensions=2  InputPortWidth=3  IndexOptions=Index vector (dialog),Index vector (dialog)  Indices=1,3  OutputSizes=1,1
  32 : Selector  NumberOfDimensions=2  InputPortWidth=3  IndexOptions=Index vector (dialog),Index vector (dialog)  Indices=3,2  OutputSizes=1,1
  33 : Selector  NumberOfDimensions=2  InputPortWidth=3  IndexOptions=Index vector (dialog),Index vector (dialog)  Indices=3,3  OutputSizes=1,1
  Gain : Gain  Gain=-1
  Product : Product
  Product1 : Product
  Subtract : Sum  Inputs=+-
  Out1 : Outport
  wires:
  In1/1 -> 32/1, 13/1, 33/1, 12/1
  12/1 -> Product/1
  33/1 -> Product/2
  13/1 -> Product1/1
  32/1 -> Product1/2
  Subtract/1 -> Gain/1
  Product/1 -> Subtract/1
  Product1/1 -> Subtract/2
  Gain/1 -> Out1/1

== system ATTITUDE_DETERMINATION/Q method/q_opt computing/Det 3x3/Adj 3x3/C22 ==
  In1 : Inport
  11 : Selector  NumberOfDimensions=2  InputPortWidth=3  IndexOptions=Index vector (dialog),Index vector (dialog)  Indices=1,1  OutputSizes=1,1
  13 : Selector  NumberOfDimensions=2  InputPortWidth=3  IndexOptions=Index vector (dialog),Index vector (dialog)  Indices=1,3  OutputSizes=1,1
  31 : Selector  NumberOfDimensions=2  InputPortWidth=3  IndexOptions=Index vector (dialog),Index vector (dialog)  Indices=3,1  OutputSizes=1,1
  33 : Selector  NumberOfDimensions=2  InputPortWidth=3  IndexOptions=Index vector (dialog),Index vector (dialog)  Indices=3,3  OutputSizes=1,1
  Product : Product
  Product1 : Product
  Subtract : Sum  Inputs=+-
  Out1 : Outport
  wires:
  In1/1 -> 31/1, 13/1, 33/1, 11/1
  11/1 -> Product/1
  33/1 -> Product/2
  13/1 -> Product1/1
  31/1 -> Product1/2
  Subtract/1 -> Out1/1
  Product/1 -> Subtract/1
  Product1/1 -> Subtract/2

== system ATTITUDE_DETERMINATION/Q method/q_opt computing/Det 3x3/Adj 3x3/C23 ==
  In1 : Inport
  11 : Selector  NumberOfDimensions=2  InputPortWidth=3  IndexOptions=Index vector (dialog),Index vector (dialog)  Indices=1,1  OutputSizes=1,1
  12 : Selector  NumberOfDimensions=2  InputPortWidth=3  IndexOptions=Index vector (dialog),Index vector (dialog)  Indices=1,2  OutputSizes=1,1
  31 : Selector  NumberOfDimensions=2  InputPortWidth=3  IndexOptions=Index vector (dialog),Index vector (dialog)  Indices=3,1  OutputSizes=1,1
  32 : Selector  NumberOfDimensions=2  InputPortWidth=3  IndexOptions=Index vector (dialog),Index vector (dialog)  Indices=3,2  OutputSizes=1,1
  Gain : Gain  Gain=-1
  Product : Product
  Product1 : Product
  Subtract : Sum  Inputs=+-
  Out1 : Outport
  wires:
  In1/1 -> 12/1, 31/1, 32/1, 11/1
  11/1 -> Product/1
  32/1 -> Product/2
  31/1 -> Product1/1
  12/1 -> Product1/2
  Subtract/1 -> Gain/1
  Product/1 -> Subtract/1
  Product1/1 -> Subtract/2
  Gain/1 -> Out1/1

== system ATTITUDE_DETERMINATION/Q method/q_opt computing/Det 3x3/Adj 3x3/C31 ==
  In1 : Inport
  12 : Selector  NumberOfDimensions=2  InputPortWidth=3  IndexOptions=Index vector (dialog),Index vector (dialog)  Indices=1,2  OutputSizes=1,1
  13 : Selector  NumberOfDimensions=2  InputPortWidth=3  IndexOptions=Index vector (dialog),Index vector (dialog)  Indices=1,3  OutputSizes=1,1
  22 : Selector  NumberOfDimensions=2  InputPortWidth=3  IndexOptions=Index vector (dialog),Index vector (dialog)  Indices=2,2  OutputSizes=1,1
  23 : Selector  NumberOfDimensions=2  InputPortWidth=3  IndexOptions=Index vector (dialog),Index vector (dialog)  Indices=2,3  OutputSizes=1,1
  Product : Product
  Product1 : Product
  Subtract : Sum  Inputs=+-
  Out1 : Outport
  wires:
  In1/1 -> 22/1, 13/1, 23/1, 12/1
  12/1 -> Product/1
  23/1 -> Product/2
  13/1 -> Product1/1
  22/1 -> Product1/2
  Subtract/1 -> Out1/1
  Product/1 -> Subtract/1
  Product1/1 -> Subtract/2

== system ATTITUDE_DETERMINATION/Q method/q_opt computing/Det 3x3/Adj 3x3/C32 ==
  In1 : Inport
  11 : Selector  NumberOfDimensions=2  InputPortWidth=3  IndexOptions=Index vector (dialog),Index vector (dialog)  Indices=1,1  OutputSizes=1,1
  13 : Selector  NumberOfDimensions=2  InputPortWidth=3  IndexOptions=Index vector (dialog),Index vector (dialog)  Indices=1,3  OutputSizes=1,1
  23 : Selector  NumberOfDimensions=2  InputPortWidth=3  IndexOptions=Index vector (dialog),Index vector (dialog)  Indices=2,3  OutputSizes=1,1
  31 : Selector  NumberOfDimensions=2  InputPortWidth=3  IndexOptions=Index vector (dialog),Index vector (dialog)  Indices=3,1  OutputSizes=1,1
  Gain : Gain  Gain=-1
  Product : Product
  Product1 : Product
  Subtract : Sum  Inputs=+-
  Out1 : Outport
  wires:
  In1/1 -> 31/1, 13/1, 23/1, 11/1
  11/1 -> Product/1
  23/1 -> Product/2
  13/1 -> Product1/1
  31/1 -> Product1/2
  Subtract/1 -> Gain/1
  Product/1 -> Subtract/1
  Product1/1 -> Subtract/2
  Gain/1 -> Out1/1

== system ATTITUDE_DETERMINATION/Q method/q_opt computing/Det 3x3/Adj 3x3/C33 ==
  In1 : Inport
  11 : Selector  NumberOfDimensions=2  InputPortWidth=3  IndexOptions=Index vector (dialog),Index vector (dialog)  Indices=1,1  OutputSizes=1,1
  12 : Selector  NumberOfDimensions=2  InputPortWidth=3  IndexOptions=Index vector (dialog),Index vector (dialog)  Indices=1,2  OutputSizes=1,1
  21 : Selector  NumberOfDimensions=2  InputPortWidth=3  IndexOptions=Index vector (dialog),Index vector (dialog)  Indices=2,1  OutputSizes=1,1
  22 : Selector  NumberOfDimensions=2  InputPortWidth=3  IndexOptions=Index vector (dialog),Index vector (dialog)  Indices=2,2  OutputSizes=1,1
  Product : Product
  Product1 : Product
  Subtract : Sum  Inputs=+-
  Out1 : Outport
  wires:
  In1/1 -> 21/1, 12/1, 22/1, 11/1
  11/1 -> Product/1
  22/1 -> Product/2
  12/1 -> Product1/1
  21/1 -> Product1/2
  Subtract/1 -> Out1/1
  Product/1 -> Subtract/1
  Product1/1 -> Subtract/2

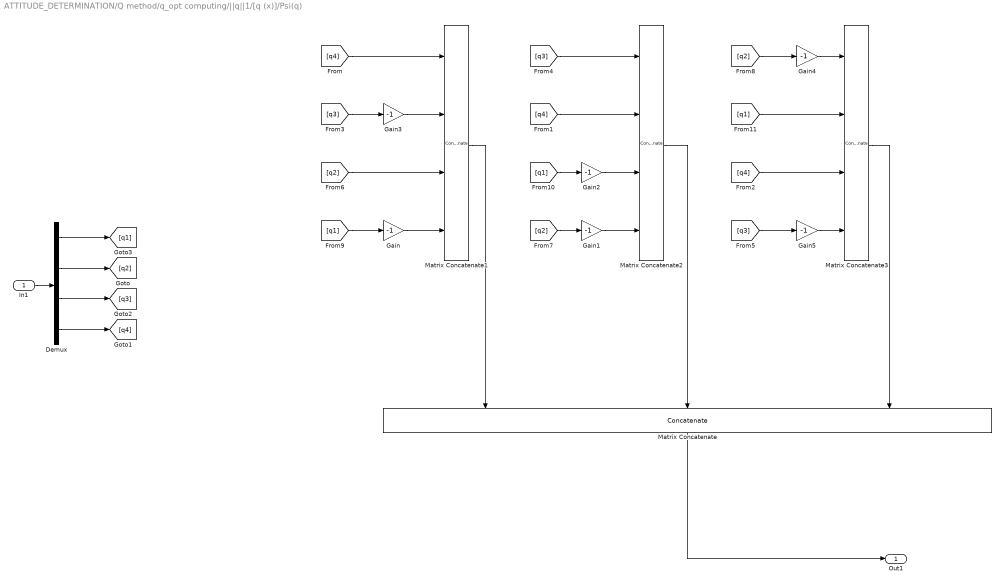
== system ATTITUDE_DETERMINATION/Q method/q_opt computing/||q||1/[q (x)]/Psi(q) ==
  In1 : Inport
  Demux : Demux
  Gain{,1..5} (6 alike) : Gain  Gain=-1
  Matrix Concatenate : Concatenate  NumInputs=3  Mode=Multidimensional array  ConcatenateDimension=2
  Matrix Concatenate1 : Concatenate  NumInputs=4  Mode=Multidimensional array
  Matrix Concatenate2 : Concatenate  NumInputs=4  Mode=Multidimensional array
  Matrix Concatenate3 : Concatenate  NumInputs=4  Mode=Multidimensional array
  Out1 : Outport
  wires:
  [q1] -> Matrix Concatenate3/2
  [q1] -> Gain2/1
  [q1] -> Gain/1
  [q2] -> Gain4/1
  [q2] -> Gain1/1
  [q2] -> Matrix Concatenate1/3
  [q3] -> Gain5/1
  [q3] -> Matrix Concatenate2/1
  [q3] -> Gain3/1
  [q4] -> Matrix Concatenate3/3
  [q4] -> Matrix Concatenate2/2
  [q4] -> Matrix Concatenate1/1
  Gain5/1 -> Matrix Concatenate3/4
  Gain4/1 -> Matrix Concatenate3/1
  Gain3/1 -> Matrix Concatenate1/2
  Gain/1 -> Matrix Concatenate1/4
  Gain2/1 -> Matrix Concatenate2/3
  Gain1/1 -> Matrix Concatenate2/4
  Matrix Concatenate3/1 -> Matrix Concatenate/3
  Matrix Concatenate2/1 -> Matrix Concatenate/2
  Matrix Concatenate1/1 -> Matrix Concatenate/1
  Matrix Concatenate/1 -> Out1/1
  Demux/1 -> [q1]
  Demux/4 -> [q4]
  Demux/3 -> [q3]
  Demux/2 -> [q2]
  In1/1 -> Demux/1
